simulink model "MySusp_Stabi_RTW"  (Simulink 9.1)
settings: Solver=ode1  StartTime=0.0  StopTime=inf  FixedStep=0.001  RelTol=1e-3
PreLoadFcn:
  | vehicle = 'Car'; if ~length(which('cmself')), cmenv; end
  | MySusp_Stabi_RTW_bus
  | MySusp_Stabi_RTW_params
InitFcn:
  | vehicle = 'Car'; if ~length(which('cmself')), cmenv; end
  | MySusp_Stabi_RTW_bus
values from neighbouring files (symbols this model uses):
  Stiffness = 50000    [MySusp_ParasiticFriction_RTW_params.m]    (also in MySusp_Spring_RTW_params.m = 5000; MySusp_Stabi_RTW_params.m = 15000)
Description:
  | CarMaker Plug-in Model Target
settings Model: SuppressorTable=22 serialization::archive 11 0 6 0 0 0 1 0  Creator=ml  LastModifiedBy=ml
settings DataIOCC: SaveFormat=Dataset
settings OptimizationCC: LifeSpan=auto
settings DebuggingCC: UnderspecifiedInitializationDetection=Simplified  MergeDetectMultiDrivingBlocksExec=error  SFUnexpectedBacktrackingDiag=error  SFNoUnconditionalDefaultTransitionDiag=error  SFExecutionAtInitializationDiag=warning
settings HardwareCC: ProdBitPerPointer=64  ProdBitPerSizeT=64  ProdBitPerPtrDiffT=64  ProdLargestAtomicFloat=Float  ProdIntDivRoundTo=Zero  ProdEndianess=LittleEndian  ProdWordSize=64  ProdHWDeviceType=Intel->x86-64 (Windows64)
settings ModelReferenceCC: PropagateSignalLabelsOutOfModel=on
settings RTWCC: SystemTargetFile=CarMaker.tlc  TemplateMakefile=CarMaker_unix-win64.tmf  Description=CarMaker Plug-in Model Target
settings CodeAppCC: MaxIdLength=127
settings STFCustomTargetCC: TargetLangStandard=C99 (ISO)  CombineOutputUpdateFcns=on  MultiInstanceERTCode=on  CodeInterfacePackaging=Reusable function  GRTInterface=off  GenerateAllocFcn=on  SystemTargetFile=CarMaker.tlc
settings GRTTargetCC: TargetLangStandard=C99 (ISO)  ParMdlRefBuildCompliant=off  CompOptLevelCompliant=off  ConcurrentExecutionCompliant=off  CombineOutputUpdateFcns=on  MatFileLogging=off  MultiInstanceERTCode=on  CodeInterfacePackaging=Reusable function  CPPClassGenCompliant=off  GRTInterface=off  GenerateAllocFcn=on  UseToolchainInfoCompliant=off  RTWCAPISignals=on  RTWCAPIParams=on  RTWCAPIStates=on
settings CustomProperty: DataType=string
settings EnumStrPairs: String=Car
settings ConfigComp: CovMetricSettings=dwe  CovHtmlReporting=off  CovSaveCumulativeToWorkspaceVar=off  CovSaveSingleToWorkspaceVar=off  CovExternalEMLEnable=on

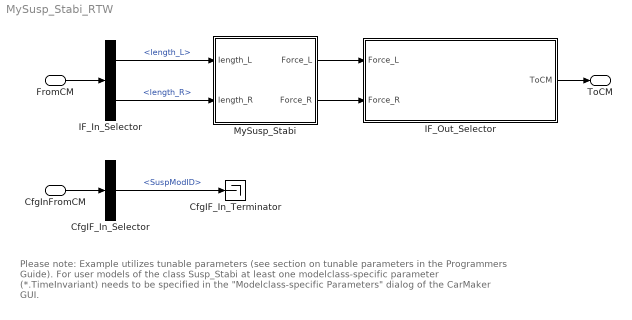
== system MySusp_Stabi_RTW ==
  note: Please note: Example utilizes tunable parameters (see section on tunable parameters in the Programmers Guide).
      |
      | For user models of the class Susp_Stabi at least one modelclass-specific parameter (*.TimeInvariant) needs to be specified in the
      | "Modelclass-specific Parameters" dialog of the CarMaker GUI.
  FromCM : Inport  OutDataTypeStr=Bus: cmSusp_StabiIn
  CfgInFromCM : Inport  Port=2  OutDataTypeStr=Bus: cmSusp_StabiCfgIn
  CfgIF_In_Selector : BusSelector  OutputSignals=SuspModID
  CfgIF_In_Terminator : Terminator
  IF_In_Selector : BusSelector  OutputSignals=length_L,length_R
  IF_Out_Selector : Subsystem  mask(Signal Selection){}
      mask help: Signal Selection Block
      settings: OpenFcn=cmSignalSelect('SignalSelection_CB',gcb)
  MySusp_Stabi : Subsystem
  ToCM : Outport  OutDataTypeStr=Bus: cmSusp_StabiOut
  wires:
  FromCM/1 -> IF_In_Selector/1
  IF_Out_Selector/1(ToCM) -> ToCM/1
  CfgInFromCM/1 -> CfgIF_In_Selector/1
  CfgIF_In_Selector/1 -> CfgIF_In_Terminator/1  "<SuspModID>"
  IF_In_Selector/1 -> MySusp_Stabi/1(Iength_L)  "<length_L>"
  IF_In_Selector/2 -> MySusp_Stabi/2(length_R)  "<length_R>"
  MySusp_Stabi/1(Force_L) -> IF_Out_Selector/1(Force_L)
  MySusp_Stabi/2(Force_R) -> IF_Out_Selector/2(Force_R)

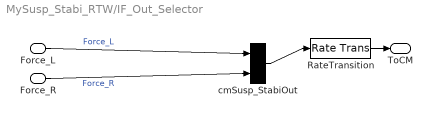
== system MySusp_Stabi_RTW/IF_Out_Selector ==
  Force_L : Inport
  Force_R : Inport  Port=2
  RateTransition : RateTransition  OutPortSampleTime=str2num(get_param(bdroot,'FixedStep'))
  cmSusp_StabiOut : BusCreator  Inputs=2
  ToCM : Outport
  wires:
  RateTransition/1 -> ToCM/1
  cmSusp_StabiOut/1 -> RateTransition/1
  Force_L/1 -> cmSusp_StabiOut/1  "Force_L"
  Force_R/1 -> cmSusp_StabiOut/2  "Force_R"

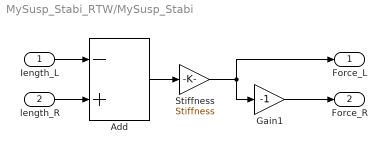
== system MySusp_Stabi_RTW/MySusp_Stabi ==
  Iength_L : Inport
  length_R : Inport  Port=2
  Add : Sum  Inputs=-+
  Gain1 : Gain  Gain=-1
  Stiffness : Gain  Gain=Stiffness
  Force_L : Outport
  Force_R : Outport  Port=2
  wires:
  Stiffness/1 -> Force_L/1, Gain1/1
  Gain1/1 -> Force_R/1
  Iength_L/1 -> Add/1
  length_R/1 -> Add/2
  Add/1 -> Stiffness/1
